simulink subsystem "rolling_resistance"  (R2024b)
settings: Solver=VariableStepAuto  StartTime=0.0  StopTime=10.0  RelTol=1e-3
settings Model: Creator=yevge  LastModifiedBy=yevge

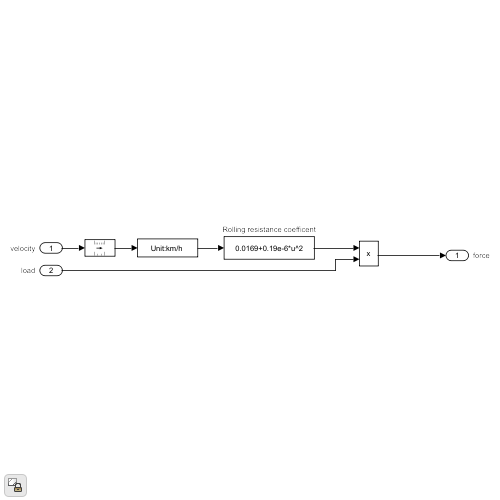
[thumbnail: Simulink's stored preview of the top-level diagram]
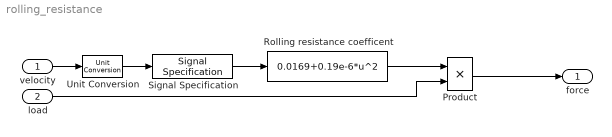
== system rolling_resistance ==
  velocity : Inport  Unit=m/s
  load : Inport  Port=2  Unit=N
  Product : Product
  Rolling resistance coefficent : Fcn  Expr=0.0169+0.19e-6*u^2
  Signal Specification : SignalSpecification  Unit=km/h
  Unit Conversion : UnitConversion
  force : Outport  Unit=N
  wires:
  load/1 -> Product/2
  Rolling resistance coefficent/1 -> Product/1
  Product/1 -> force/1
  velocity/1 -> Unit Conversion/1
  Unit Conversion/1 -> Signal Specification/1
  Signal Specification/1 -> Rolling resistance coefficent/1
